simulink model "DC_MOTOR_Paramters"  (R2018a)
settings: Solver=VariableStepAuto  StartTime=0.0  StopTime=35  RelTol=1e-3
model workspace (MAT data in the model file):
  B = 2.69254913662e-19
  J = 0.000262842480729
  K = 0.01323780842
  L = 0.00192532731313
  R = 0.08
libraries: simulink_extras x2
settings Model: Creator=Hazem Elwakeel  LastModifiedBy=Hazem Elwakeel

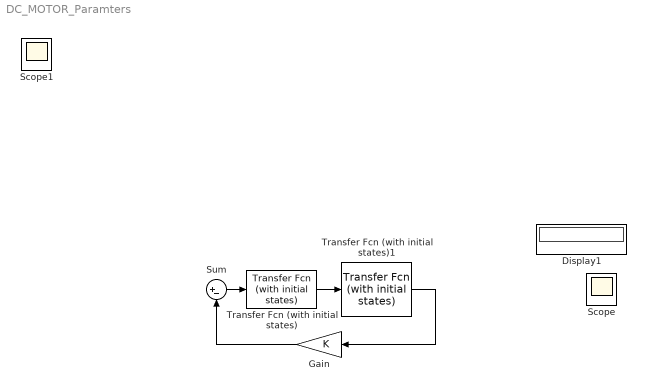
== system DC_MOTOR_Paramters ==
  Display1 : Display
  Gain : Gain  Gain=K
  Scope : Scope
  Sum : Sum  Inputs=|+-
  Transfer Fcn (with initial states) : simulink_extras/Additional Linear/Transfer Fcn (with initial states)  N=[K]  D="[J  B]"  X0=.5
  Transfer Fcn (with initial states)1 : simulink_extras/Additional Linear/Transfer Fcn (with initial states)  N=[1]  D="[L  R]"  X0=.5
  Scope1 : Scope
  wires:
  Transfer Fcn (with initial states)/1 -> Transfer Fcn (with initial states)1/1
  Sum/1 -> Transfer Fcn (with initial states)/1
  Gain/1 -> Sum/2
  Transfer Fcn (with initial states)1/1 -> Gain/1
